simulink model "rtwdemo_forloop"  (Simulink 7.6)
settings: Solver=ode5  StartTime=0.0  StopTime=10.0  FixedStep=1  RelTol=1e-3
libraries: rtwdemowidgets x2
Description:
  | For-Loop Fusion
settings Model: Creator=The MathWorks Inc.  ExtModeAutoUpdateStatusClock=off
settings MATStruct: SampleTime=1  Offset=0  Priority=[20.0]
settings DataIOCC: SaveFormat=StructureWithTime  SaveOutput=off  SaveTime=off  SignalLoggingName=sigsOut
settings OptimizationCC: InlineParams=on  UseIntDivNetSlope=on  InlineInvariantSignals=on  EnhancedBackFolding=on  StateBitsets=on  DataBitsets=on  UseTempVars=on  EfficientFloat2IntCast=on
settings DebuggingCC: CheckExecutionContextPreStartOutputMsg=on  CheckExecutionContextRuntimeOutputMsg=on  SolverPrmCheckMsg=none  StrictBusMsg=ErrorOnBusTreatedAsVector
settings HardwareCC: ProdBitPerLong=64  ProdIntDivRoundTo=Zero  ProdEndianess=LittleEndian  ProdWordSize=64  ProdHWDeviceType=Specified  TargetHWDeviceType=Generic->32-bit Embedded Processor
settings SFSimCC: SimParseCustomCode=off
settings RTWCC: TLCOptions=-p0 -aWarnNonSaturatedBlocks=0  GenerateReport=on  RTWVerbose=off  ProcessScript=grt_make_rtw_hook  LaunchReport=on
settings CodeAppCC: ForceParamTrailComments=on

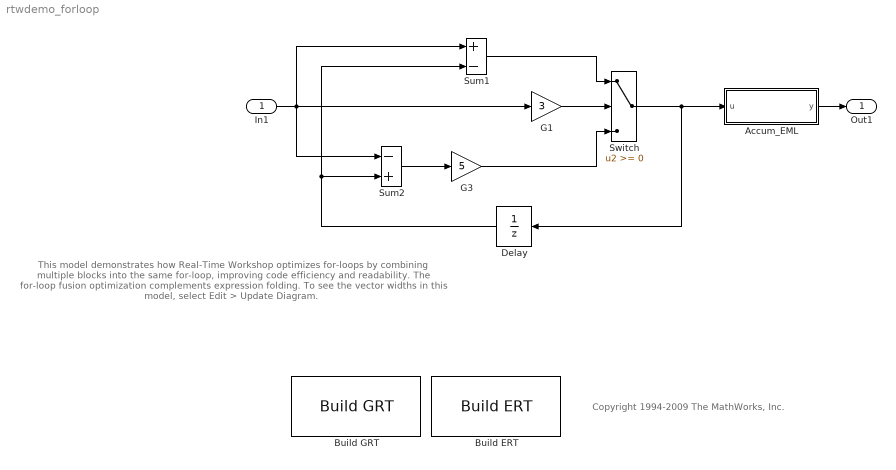
== system rtwdemo_forloop ==
  note: This model demonstrates how Real-Time Workshop optimizes for-loops by combining
      | multiple blocks into the same for-loop, improving code efficiency and readability.
      | The for-loop fusion optimization complements expression folding.  To see the vector
      | widths in this model, select Edit > Update Diagram.
  note: Copyright 1994-2009 The MathWorks, Inc.
  In1 : Inport  OutDataTypeStr=double  PortDimensions=10  SampleTime=1
  Accum_EML : Stateflow chart  TreatAsAtomicUnit=on
  Build ERT : rtwdemowidgets/Build ERT  SystemSampleTime=-1  attrib_overrides={}
  Build GRT : rtwdemowidgets/Build GRT  SystemSampleTime=-1  attrib_overrides={}
  Delay : UnitDelay
  G1 : Gain  Gain=3  SaturateOnIntegerOverflow=on  OutDataTypeStr=Inherit: Same as input  ParamDataTypeStr=Inherit: Same as input
  G3 : Gain  Gain=5  SaturateOnIntegerOverflow=on  OutDataTypeStr=Inherit: Same as input  ParamDataTypeStr=Inherit: Same as input
  Sum1 : Sum  Inputs=+-  SaturateOnIntegerOverflow=on  InputSameDT=on  OutDataTypeStr=Inherit: Same as first input
  Sum2 : Sum  Inputs=-+  SaturateOnIntegerOverflow=on  InputSameDT=on  OutDataTypeStr=Inherit: Same as first input
  Switch : Switch  ZeroCross=off  SaturateOnIntegerOverflow=on  InputSameDT=on
  Out1 : Outport
  wires:
  Sum1/1 -> Switch/1
  G1/1 -> Switch/2
  Sum2/1 -> G3/1
  Switch/1 -> Delay/1, Accum_EML/1(u)
  Delay/1 -> Sum2/2, Sum1/2
  In1/1 -> G1/1, Sum1/1, Sum2/1
  G3/1 -> Switch/3
  Accum_EML/1(y) -> Out1/1

== matlab function Accum_EML ==
  data: u input double; y output double
function y = Accum_EML(u)

a = u' + (1:10);
y = 0;
for k = 1:numel(a)
    y = y + a(k);
end
